simulink model "file6"  (R2024b)
settings: Solver=VariableStepAuto  StartTime=0.0  StopTime=10  RelTol=1e-3
InitFcn:
  | Voc=32.9;
  | Iscn=8.21;
  | k=1.38e-23;
  | NS=54;
  | Np=1;
  | Gn=1000;
  | Kv=-0.123;
  | K1=0.0032;
  | T=301;
  | Tn=300;
  | q=1.6e-19;
  | I0n=9.85e-8;
  | Eg=1.12;
  | Ign=8.214;
  | Rs=0.221;
  | Rp=414.5;
  | a=1.0;
libraries: spsSeriesRLCBranchLib x6, spsVoltageMeasurementLib x4, spsCurrentMeasurementLib x2, spsDiodeLib x2, spsMeanLib x2, spsFirstOrderFilterLib x2, spsMosfetLib x1, spsControlledCurrentSourceLib x1, simulink x1, spsPWMGeneratorDCDCLib x1, slpidlib x1, sps_lib x1
settings Model: Creator=cdsl07  LastModifiedBy=cdsl07

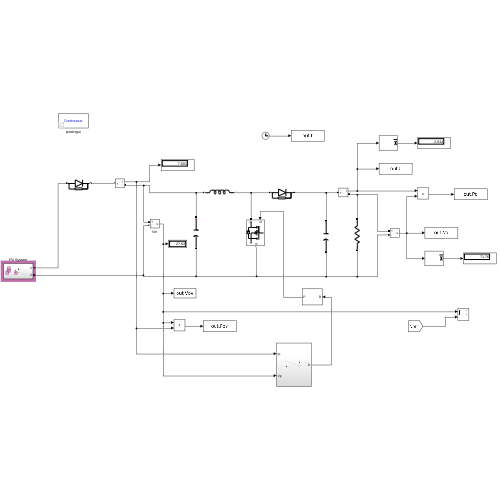
[thumbnail: Simulink's stored preview of the top-level diagram]
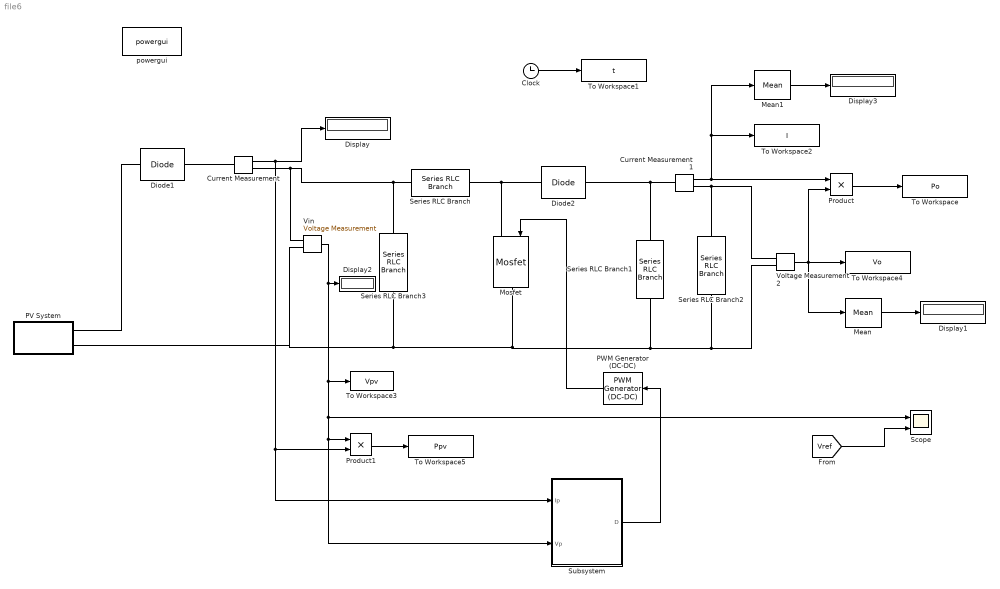
== system file6 ==
  Clock : Clock
  Current Measurement : spsCurrentMeasurementLib/Current Measurement  PhasorSimulation=off  OutputType=Complex  PSBequivalent=0
  Current Measurement1 : spsCurrentMeasurementLib/Current Measurement  PhasorSimulation=off  OutputType=Complex  PSBequivalent=0
  Diode1 : spsDiodeLib/Diode  Ron=0.001  Lon=0  Vf=0.8  IC=0  UseSnubber=0  Rs=500  Cs=250e-9  Measurements=off
  Diode2 : spsDiodeLib/Diode  Ron=0.001  Lon=0  Vf=0.8  IC=0  UseSnubber=0  Rs=500  Cs=250e-9  Measurements=off
  Display{,1..3} (4 alike) : Display
  Mean : spsMeanLib/Mean  Freq=60  Vinit=0  Ts=0
  Mean1 : spsMeanLib/Mean  Freq=60  Vinit=0  Ts=0
  Mosfet : spsMosfetLib/Mosfet  Ron=0.1  Lon=0  Rd=0.01  Vfd=0  IC=0  Rs=1e5  Cs=inf  Measurements=off
  PV System : Subsystem
  PWM Generator (DC-DC) : spsPWMGeneratorDCDCLib/PWM Generator (DC-DC)  Fsw=5e+3  Ts=0
  Product : Product
  Product1 : Product
  Scope : Scope  NumInputPorts=2
  Series RLC Branch : spsSeriesRLCBranchLib/Series RLC Branch  LConnTagsString=__new0  RConnTagsString=__new0  BranchType=L  Resistance=1  Inductance=0.01025  SetiL0=off  InitialCurrent=0  Capacitance=1e-6  Setx0=off  InitialVoltage=0  Measurements=None
  Series RLC Branch1 : spsSeriesRLCBranchLib/Series RLC Branch  LConnTagsString=__new0  RConnTagsString=__new0  BranchType=C  Resistance=1  Inductance=1e-3  SetiL0=off  InitialCurrent=0  Capacitance=110e-6  Setx0=off  InitialVoltage=0  Measurements=None
  Series RLC Branch2 : spsSeriesRLCBranchLib/Series RLC Branch  LConnTagsString=__new0  RConnTagsString=__new0  BranchType=R  Resistance=25.5  Inductance=1e-3  SetiL0=off  InitialCurrent=0  Capacitance=1e-6  Setx0=off  InitialVoltage=0  Measurements=None
  Series RLC Branch3 : spsSeriesRLCBranchLib/Series RLC Branch  LConnTagsString=__new0  RConnTagsString=__new0  BranchType=C  Resistance=1  Inductance=1e-3  SetiL0=off  InitialCurrent=0  Capacitance=110e-6  Setx0=off  InitialVoltage=0  Measurements=None
  Subsystem : Subsystem
  To Workspace : ToWorkspace  VariableName=Po  SampleTime=-1
  To Workspace1 : ToWorkspace  VariableName=t  SampleTime=-1
  To Workspace2 : ToWorkspace  VariableName=I  SampleTime=-1
  To Workspace3 : ToWorkspace  VariableName=Vpv  SampleTime=-1
  To Workspace4 : ToWorkspace  VariableName=Vo  SampleTime=-1
  To Workspace5 : ToWorkspace  VariableName=Ppv  SampleTime=-1
  Vin : spsVoltageMeasurementLib/Voltage Measurement  PhasorSimulation=off  OutputType=Complex  PSBequivalent=0
  Voltage Measurement2 : spsVoltageMeasurementLib/Voltage Measurement  PhasorSimulation=off  OutputType=Complex  PSBequivalent=0
  powergui : sps_lib/powergui  Priority=1  SimulationMode=Continuous  SampleTime=50e-6  frequency=60  Iterations=50  frequencyindice=0  Pbase=100e6  ErrMax=1e-4  UnitsV=kV  UnitsW=MW  buscounter=0  FunctionMessages=off  echomessages=off  EnableUseOfTLC=off  CurrentSourceSwitches=off  DisableSnubberDevices=off  DisableRonSwitches=off  DisableVfSwitches=off  DisplayEquations=off  AutomaticDiscreteSolvers=off  SolverType=Tustin/Backward Euler (TBE)  Interpol=off  ExternalGateDelay=off  methode=off  Ts=100  x0status=blocks  SPID=on  SwTol=0  HookPort=off  NonlinearTolerance=1e-4  nMaxIteration=100  ContinueOnMaxIteration=off  RestoreLinks=warning  ResistiveCurrentMeasurement=off  Frange=[0:2:500]  Ylog=off  Xlog=on  ShowGrid=off  save=off  variable=ZData  structure=0  ZoomFFT=off  StartTime=0.0  cycles=1  DisplayStyle=1  fundamental=60  FreqAxis=off  MaxFrequency=1000  frequencyindicesteady=1  RmsSteady=1  display=off
  wires:
  Current Measurement1/1 -> Mean1/1, To Workspace2/1, Product/1
  Product/1 -> To Workspace/1
  Voltage Measurement2/1 -> Mean/1, Product/2, To Workspace4/1
  Mean/1 -> Display1/1
  Clock/1 -> To Workspace1/1
  Mean1/1 -> Display3/1
  Current Measurement/1 -> Subsystem/1(Ip), Product1/2, Display/1
  Vin/1 -> Subsystem/2(Vp), Product1/1, Scope/1, To Workspace3/1, Display2/1
  Subsystem/1(D) -> PWM Generator (DC-DC)/1
  Product1/1 -> To Workspace5/1
  PWM Generator (DC-DC)/1 -> Mosfet/1
  [Vref] -> Scope/2
  connections:
  Current Measurement1/LConn1 -- Diode2/RConn1 -- Series RLC Branch1/LConn1
  Series RLC Branch1/RConn1 -- Vin/LConn2 -- PV System/LConn2 -- Series RLC Branch3/RConn1 -- Mosfet/RConn1 -- Voltage Measurement2/LConn2 -- Series RLC Branch2/RConn1
  Series RLC Branch/LConn1 -- Vin/LConn1 -- Current Measurement/RConn1 -- Series RLC Branch3/LConn1
  Diode1/RConn1 -- Current Measurement/LConn1
  Diode1/LConn1 -- PV System/LConn1
  Current Measurement1/RConn1 -- Voltage Measurement2/LConn1 -- Series RLC Branch2/LConn1
  Series RLC Branch/RConn1 -- Mosfet/LConn1 -- Diode2/LConn1

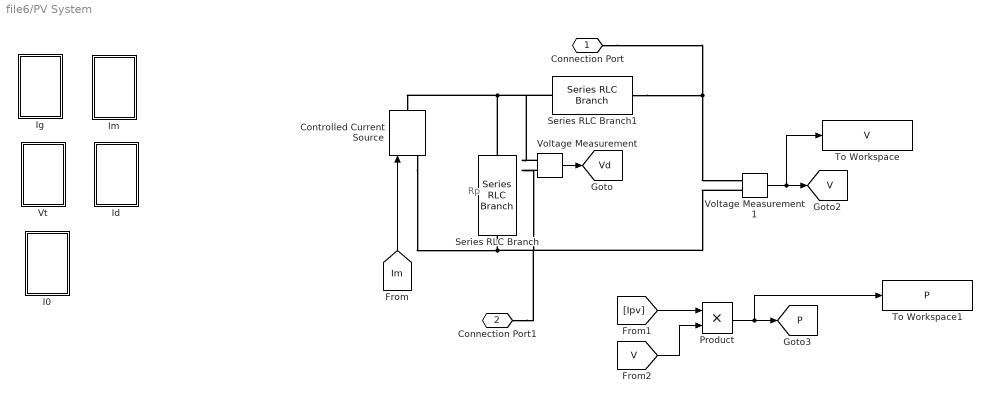
== system file6/PV System ==
  note: Rp
  Controlled Current Source : spsControlledCurrentSourceLib/Controlled Current Source  Initialize=on  Source_Type=AC  Amplitude=0  Phase=0  Frequency=0  Measurements=None
  I0 : Subsystem
  Id : Subsystem
  Ig : Subsystem
  Im : Subsystem
  Product : Product
  Series RLC Branch : spsSeriesRLCBranchLib/Series RLC Branch  LConnTagsString=__new0  RConnTagsString=__new0  BranchType=R  Resistance=Rp  Inductance=1e-3  SetiL0=off  InitialCurrent=0  Capacitance=1e-6  Setx0=off  InitialVoltage=0  Measurements=None
  Series RLC Branch1 : spsSeriesRLCBranchLib/Series RLC Branch  LConnTagsString=__new0  RConnTagsString=__new0  BranchType=R  Resistance=Rs  Inductance=1e-3  SetiL0=off  InitialCurrent=0  Capacitance=1e-6  Setx0=off  InitialVoltage=0  Measurements=None
  To Workspace : ToWorkspace  VariableName=V  SampleTime=-1
  To Workspace1 : ToWorkspace  VariableName=P  SampleTime=-1
  Voltage Measurement : spsVoltageMeasurementLib/Voltage Measurement  PhasorSimulation=off  OutputType=Complex  PSBequivalent=0
  Voltage Measurement1 : spsVoltageMeasurementLib/Voltage Measurement  PhasorSimulation=off  OutputType=Complex  PSBequivalent=0
  Vt : Subsystem
  Connection Port : PMIOPort  Side=Left
  Connection Port1 : PMIOPort  Port=2  Side=Left
  tag scope: P=global, V=global, Vd=global
  wires:
  Voltage Measurement1/1 -> To Workspace/1, [V]
  [Ipv] -> Product/1
  [Im] -> Controlled Current Source/1
  [V] -> Product/2
  Product/1 -> To Workspace1/1, [P]
  Voltage Measurement/1 -> [Vd]
  connections:
  Controlled Current Source/LConn1 -- Connection Port1/RConn1 -- Voltage Measurement1/LConn2 -- Voltage Measurement/LConn2 -- Series RLC Branch/LConn1
  Series RLC Branch/RConn1 -- Voltage Measurement/LConn1 -- Series RLC Branch1/LConn1 -- Controlled Current Source/RConn1
  Series RLC Branch1/RConn1 -- Connection Port/RConn1 -- Voltage Measurement1/LConn1

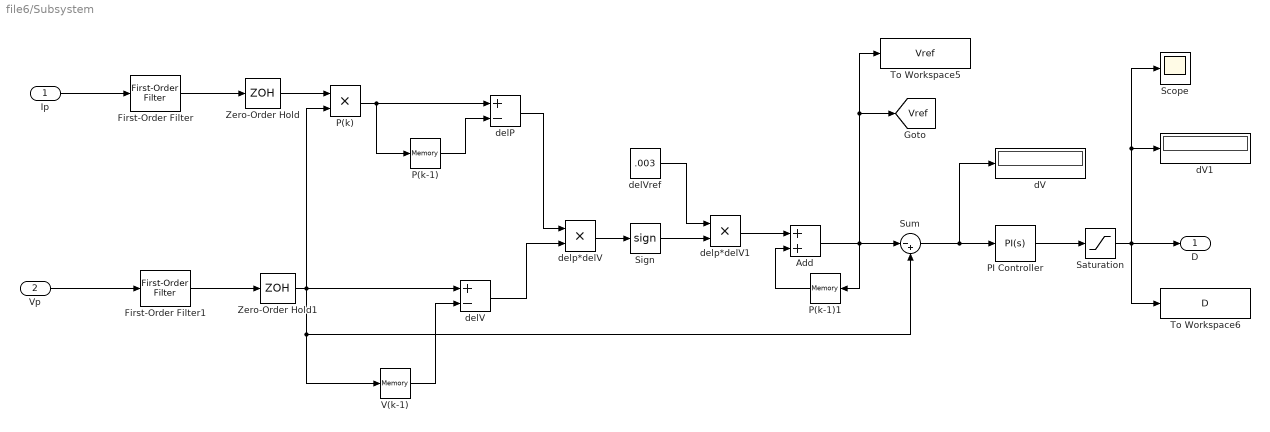
== system file6/Subsystem ==
  Ip : Inport
  Vp : Inport  Port=2
  Add : Sum
  First-Order Filter : spsFirstOrderFilterLib/First-Order Filter  FilterType=Lowpass  Tc=10e-3  Ts=0  Initialize=on  Vac_Init=[0, 0, 60]  Vdc_Init=0  PlotResponse=off  FreqRange="[0,  200,  1]"
  First-Order Filter1 : spsFirstOrderFilterLib/First-Order Filter  FilterType=Lowpass  Tc=10e-3  Ts=0  Initialize=on  Vac_Init=[0, 0, 60]  Vdc_Init=0  PlotResponse=off  FreqRange="[0,  200,  1]"
  P(k) : Product
  P(k-1) : Memory
  P(k-1)1 : Memory
  PI Controller : slpidlib/PID Controller  Controller=PI  Form=Parallel  TimeDomain=Continuous-time  UseExternalTs=off  SampleTime=-1  IntegratorMethod=Forward Euler  FilterMethod=Forward Euler  ControllerParametersSource=internal  P=0.001  I=0.1  UseKiTs=off  D=0  UseExternalDerivativeSource=off  N=100  UseFilter=on  TunerSelectOption=Transfer Function Based (PID Tuner App)  InitialConditionSource=internal  InitialConditionForIntegrator=0  InitialConditionForFilter=0  DifferentiatorICPrevScaledInput=0  ExternalReset=none  TrackingMode=off  Kt=1  LimitOutput=off  SatLimitsSource=internal  UpperSaturationLimit=inf  LowerSaturationLimit=-inf  LinearizeAsGain=on  AntiWindupMode=none  Kb=1  LimitIntegrator=off  UpperIntegratorSaturationLimit=inf  LowerIntegratorSaturationLimit=-inf  POutMin=[]  POutMax=[]  IOutMin=[]  IOutMax=[]  DOutMin=[]  DOutMax=[]  NOutMin=[]  NOutMax=[]  SumOutMin=[]  SumOutMax=[]  SaturationOutMin=[]  SaturationOutMax=[]  PParamMin=[]  PParamMax=[]  IParamMin=[]  IParamMax=[]  DParamMin=[]  DParamMax=[]  NParamMin=[]  NParamMax=[]  KbParamMin=[]  KbParamMax=[]  KtParamMin=[]  KtParamMax=[]  KbOutMin=[]  KbOutMax=[]  KtOutMin=[]  KtOutMax=[]  IntegratorOutMin=[]  IntegratorOutMax=[]  FilterOutMin=[]  FilterOutMax=[]  SumI1OutMin=[]  SumI1OutMax=[]  SumI2OutMin=[]  SumI2OutMax=[]  SumI3OutMin=[]  SumI3OutMax=[]  SumI4OutMin=[]  SumI4OutMax=[]  SumDOutMin=[]  SumDOutMax=[]  DifferentiatorOutMin=[]  DifferentiatorOutMax=[]  FilterDiffOutCoefMin=[]  FilterDiffOutCoefMax=[]  ReciprocalOutMin=[]  ReciprocalOutMax=[]  SumDenOutMin=[]  SumDenOutMax=[]  SumNumOutMin=[]  SumNumOutMax=[]  DivideOutMin=[]  DivideOutMax=[]  UdiffTsProdOutMin=[]  UdiffTsProdOutMax=[]  NTsProdOutMin=[]  NTsProdOutMax=[]  UintegralTsProdOutMin=[]  UintegralTsProdOutMax=[]  UngainTsProdOutMin=[]  UngainTsProdOutMax=[]  ClampingZeroOutDataTypeStr=Inherit: Inherit via back propagation  ClampingZeroOutMin=[]  ClampingZeroOutMax=[]  FilterDenConstantOutDataTypeStr=Inherit: Inherit via back propagation  FilterDenConstantOutMin=[]  FilterDenConstantOutMax=[]  PCopyOutDataTypeStr=Inherit: Inherit via back propagation  PCopyOutMin=[]  PCopyOutMax=[]  NCopyOutDataTypeStr=Inherit: Inherit via back propagation  NCopyOutMin=[]  NCopyOutMax=[]  IntegratorContinuousStateAttributes=''  IntegratorStateMustResolveToSignalObject=off  IntegratorRTWStateStorageClass=Auto  FilterContinuousStateAttributes=''  FilterStateMustResolveToSignalObject=off  FilterRTWStateStorageClass=Auto  ParallelPVariant=InternalParameters  IdealPVariant=Disabled  IVariant=InternalParameters  DVariant=Disabled  IntegratorVariant=Continuous  SatVariant=Disabled  AWVariant=Passthrough  PCopyVariant=Disabled  TRVariant=Disabled  FdbkBlocksVariant=Forward  IdealPFdbkVariant=Disabled  SatFdbkVariant=Disabled  DerivativeFilterVariant=Disabled  NVariant=Disabled  NCopyVariant=Disabled_SignalSpec  FilterICVariant=Disabled  IntegratorICVariant=InternalICs  ExternalResetVariant=Disabled  TRSumVariant=Passthrough  SumFdbkVariant=Disabled  SumVariant=Sum_PI  TsampFilterVariant=InternalTs  TsampNgainVariant=Passthrough  TsampIntegralVariant=Disabled_SignalSpec  ExternalSaturationOutDataTypeStr=Inherit: Same as second input  DerivativeSourceVariant=Disabled  PreIntVariant=InternalPreInt
  Saturation : Saturate  UpperLimit=1  LowerLimit=0
  Scope : Scope
  Sign : Signum
  Sum : Sum  Inputs=|-+
  To Workspace5 : ToWorkspace  VariableName=Vref  SampleTime=-1
  To Workspace6 : ToWorkspace  VariableName=D  SampleTime=-1
  V(k-1) : Memory
  Zero-Order Hold : ZeroOrderHold  SampleTime=0.0001
  Zero-Order Hold1 : ZeroOrderHold  SampleTime=0.0001
  dV : Display
  dV1 : Display
  delP : Sum  Inputs=+-
  delV : Sum  Inputs=+-
  delVref : Constant  Value=.003
  delp*delV : Product
  delp*delV1 : Product
  D : Outport
  tag scope: Vref=global
  wires:
  Zero-Order Hold/1 -> P(k)/1
  P(k-1)/1 -> delP/2
  Sum/1 -> dV/1, PI Controller/1
  Add/1 -> P(k-1)1/1, Sum/1, To Workspace5/1, [Vref]
  First-Order Filter/1 -> Zero-Order Hold/1
  First-Order Filter1/1 -> Zero-Order Hold1/1
  P(k-1)1/1 -> Add/2
  Saturation/1 -> D/1, To Workspace6/1, dV1/1, Scope/1
  P(k)/1 -> P(k-1)/1, delP/1
  delVref/1 -> delp*delV1/1
  Zero-Order Hold1/1 -> Sum/2, V(k-1)/1, delV/1, P(k)/2
  Vp/1 -> First-Order Filter1/1
  delP/1 -> delp*delV/1
  Ip/1 -> First-Order Filter/1
  delp*delV/1 -> Sign/1
  PI Controller/1 -> Saturation/1
  delV/1 -> delp*delV/2
  V(k-1)/1 -> delV/2
  Sign/1 -> delp*delV1/2
  delp*delV1/1 -> Add/1

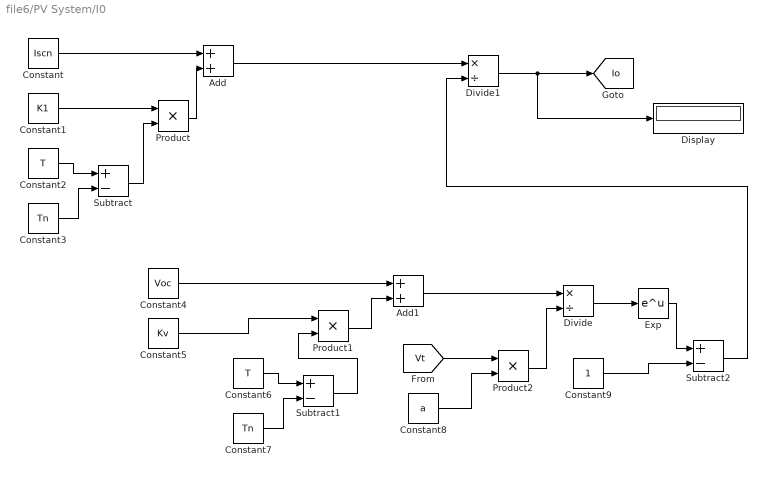
== system file6/PV System/I0 ==
  Add : Sum
  Add1 : Sum
  Constant : Constant  Value=Iscn
  Constant1 : Constant  Value=K1
  Constant2 : Constant  Value=T
  Constant3 : Constant  Value=Tn
  Constant4 : Constant  Value=Voc
  Constant5 : Constant  Value=Kv
  Constant6 : Constant  Value=T
  Constant7 : Constant  Value=Tn
  Constant8 : Constant  Value=a
  Constant9 : Constant
  Display : Display
  Divide : Product  Inputs=*/
  Divide1 : Product  Inputs=*/
  Exp : Math
  Product : Product
  Product1 : Product
  Product2 : Product
  Subtract : Sum  Inputs=+-
  Subtract1 : Sum  Inputs=+-
  Subtract2 : Sum  Inputs=+-
  tag scope: Io=global
  wires:
  Constant4/1 -> Add1/1
  Subtract1/1 -> Product1/2
  Constant1/1 -> Product/1
  Constant/1 -> Add/1
  Subtract2/1 -> Divide1/2
  [Vt] -> Product2/1
  Add/1 -> Divide1/1
  Product1/1 -> Add1/2
  Divide/1 -> Exp/1
  Divide1/1 -> Display/1, [Io]
  Constant7/1 -> Subtract1/2
  Product2/1 -> Divide/2
  Subtract/1 -> Product/2
  Constant2/1 -> Subtract/1
  Constant6/1 -> Subtract1/1
  Constant9/1 -> Subtract2/2
  Constant5/1 -> Product1/1
  Constant8/1 -> Product2/2
  Product/1 -> Add/2
  Constant3/1 -> Subtract/2
  Exp/1 -> Subtract2/1
  Add1/1 -> Divide/1

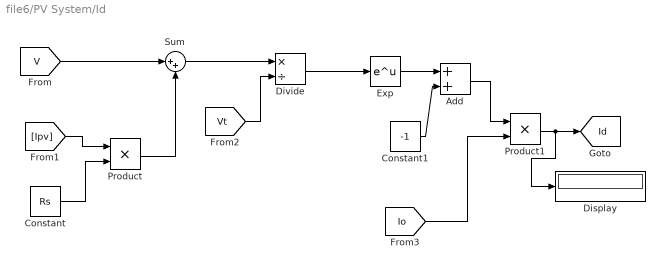
== system file6/PV System/Id ==
  Add : Sum
  Constant : Constant  Value=Rs
  Constant1 : Constant  Value=-1
  Display : Display
  Divide : Product  Inputs=*/
  Exp : Math
  Product : Product
  Product1 : Product
  Sum : Sum  Inputs=|++
  tag scope: Id=global
  wires:
  [Ipv] -> Product/1
  Product1/1 -> Display/1, [Id]
  [Io] -> Product1/2
  Sum/1 -> Divide/1
  [Vt] -> Divide/2
  Product/1 -> Sum/2
  Constant1/1 -> Add/2
  [V] -> Sum/1
  Exp/1 -> Add/1
  Constant/1 -> Product/2
  Add/1 -> Product1/1
  Divide/1 -> Exp/1

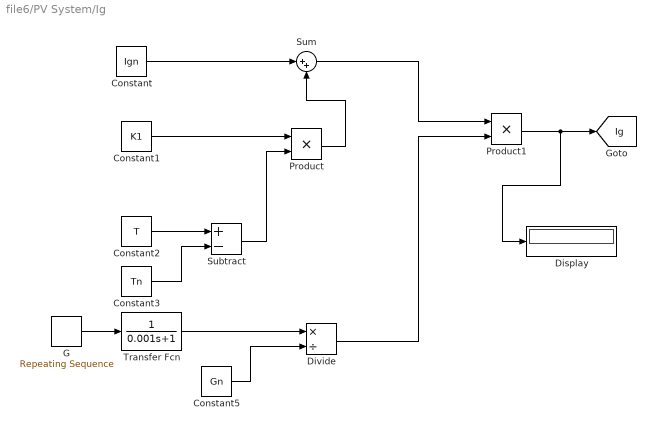
== system file6/PV System/Ig ==
  Constant : Constant  Value=Ign
  Constant1 : Constant  Value=K1
  Constant2 : Constant  Value=T
  Constant3 : Constant  Value=Tn
  Constant5 : Constant  Value=Gn
  Display : Display
  Divide : Product  Inputs=*/
  G : simulink/Sources/Repeating Sequence  rep_seq_t=[0 3 3.1 7 7.1 10]  rep_seq_y=[640 640 810 810 980 980]
  Product : Product
  Product1 : Product
  Subtract : Sum  Inputs=+-
  Sum : Sum  Inputs=|++
  Transfer Fcn : TransferFcn  Denominator=[0.001 1]
  tag scope: Ig=global
  wires:
  Product/1 -> Sum/2
  Constant2/1 -> Subtract/1
  Constant/1 -> Sum/1
  Constant5/1 -> Divide/2
  Constant3/1 -> Subtract/2
  Divide/1 -> Product1/2
  Product1/1 -> Display/1, [Ig]
  Subtract/1 -> Product/2
  Sum/1 -> Product1/1
  Constant1/1 -> Product/1
  G/1 -> Transfer Fcn/1
  Transfer Fcn/1 -> Divide/1

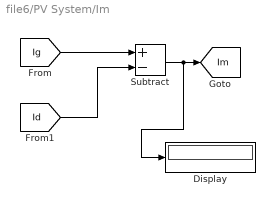
== system file6/PV System/Im ==
  Display : Display
  Subtract : Sum  Inputs=+-
  tag scope: Im=global
  wires:
  [Ig] -> Subtract/1
  [Id] -> Subtract/2
  Subtract/1 -> Display/1, [Im]

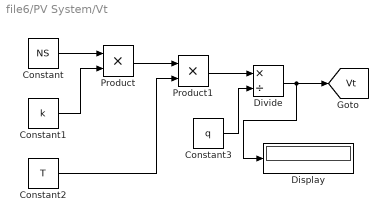
== system file6/PV System/Vt ==
  Constant : Constant  Value=NS
  Constant1 : Constant  Value=k
  Constant2 : Constant  Value=T
  Constant3 : Constant  Value=q
  Display : Display
  Divide : Product  Inputs=*/
  Product : Product
  Product1 : Product
  tag scope: Vt=global
  wires:
  Constant3/1 -> Divide/2
  Constant2/1 -> Product1/2
  Product1/1 -> Divide/1
  Product/1 -> Product1/1
  Constant/1 -> Product/1
  Constant1/1 -> Product/2
  Divide/1 -> Display/1, [Vt]
